simulink model "Controllo_assex_Rigido"  (R2020b)
settings: Solver=VariableStepAuto  StartTime=0.0  StopTime=5  RelTol=1e-3
values from neighbouring files (symbols this model uses):
  m = config_dc(parx)    [main.m]
  parx = parametri()    [main.m]
undefined symbols (not defined in the file or in its folder): Evaluate_Trajectory
libraries: cstblocks x2
settings Model: Creator=stefa  LastModifiedBy=user
settings DebuggingCC: AlgebraicLoopMsg=none  SFMachineParentedDataDiag=error

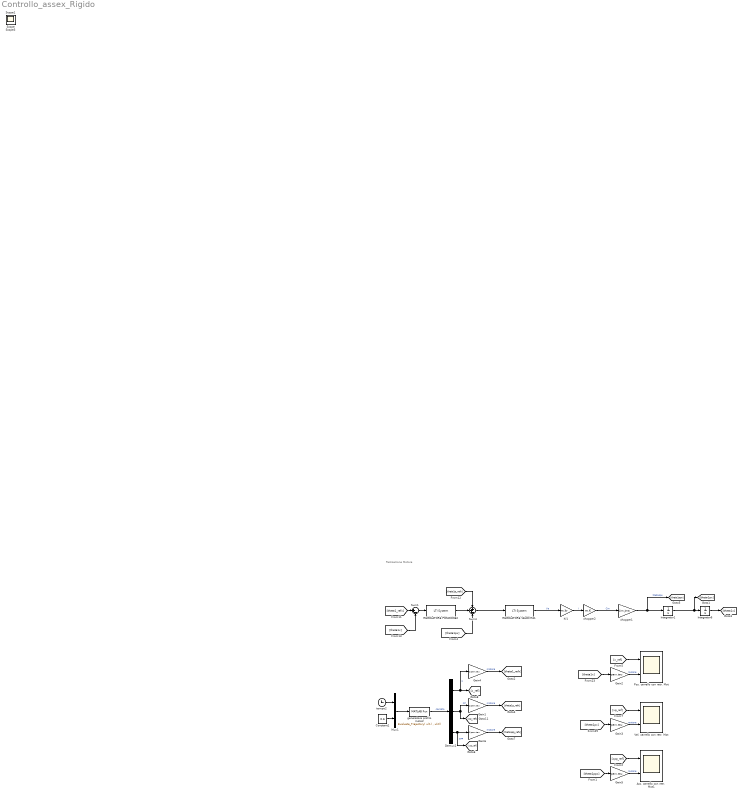
== system Controllo_assex_Rigido ==
  note: Retroazione Motore
  Acc. carrello con retr. Mot1 : Scope  NumInputPorts=2
  Constant1 : Constant  Value=0.6
  Demux2 : Demux  Outputs=3
  Gain1 : Gain  Gain=1/parx.tau
  Gain2 : Gain  Gain=parx.tau
  Gain3 : Gain  Gain=parx.tau
  Gain4 : Gain  Gain=1/parx.tau
  Gain5 : Gain  Gain=parx.tau
  Gain6 : Gain  Gain=1/parx.tau
  Integrator1 : Integrator
  Integrator6 : Integrator
  Kr1 : Gain  Gain=m.kr
  Mux1 : Mux  Inputs=2
  Pos. carrello con retr. Mot : Scope  NumInputPorts=2
  REGOLATORE POSIZIONE2 : cstblocks/LTI System  sys=ap.H_P  IC=[]
  REGOLATORE VELOCITA1 : cstblocks/LTI System  sys=av.PI_V  IC=[]
  Sum1 : Sum  Inputs=|+-
  Sum4 : Sum  Inputs=++-
  Vel. carrello con retr. Mot : Scope  NumInputPorts=2
  chopper1 : Gain  Gain=1/m.Jma
  chopper2 : Gain  Gain=m.K
  generatore profilo moto2 : MATLABFcn  MATLABFcn=Evaluate_Trajectory( u(1) , u(2))  OutputDimensions=3
  tempo2 : Clock
  Scope : Scope
  Scope1 : Scope
  Scope3 : Scope
  wires:
  Mux1/1 -> generatore profilo moto2/1
  generatore profilo moto2/1 -> Demux2/1  "carrello"
  Constant1/1 -> Mux1/2
  tempo2/1 -> Mux1/1
  Demux2/1 -> [x_ref], Gain4/1  "X"
  Demux2/2 -> Gain1/1, [xp_ref]  "XP"
  Kr1/1 -> chopper2/1  "I"
  Sum1/1 -> REGOLATORE POSIZIONE2/1
  REGOLATORE POSIZIONE2/1 -> Sum4/2
  REGOLATORE VELOCITA1/1 -> Kr1/1  "Va"
  [xp_ref] -> Vel. carrello con retr. Mot/1
  Sum4/1 -> REGOLATORE VELOCITA1/1
  [x_ref] -> Pos. carrello con retr. Mot/1
  [theta1p_refx] -> Sum4/1
  [theta1_refx] -> Sum1/1
  [theta1px] -> Sum4/3
  [theta1x] -> Sum1/2
  Gain1/1 -> [theta1p_refx]  "motore"
  Gain4/1 -> [theta1_refx]  "motore"
  chopper2/1 -> chopper1/1  "Cm"
  [theta1x] -> Gain2/1
  [theta1px] -> Gain3/1
  Gain3/1 -> Vel. carrello con retr. Mot/2  "motore"
  Gain2/1 -> Pos. carrello con retr. Mot/2  "motore"
  Integrator6/1 -> [theta1x]
  chopper1/1 -> [theta1ppx], Integrator1/1  "theta1px"
  Integrator1/1 -> [theta1px], Integrator6/1
  [theta1ppx] -> Gain5/1
  Gain5/1 -> Acc. carrello con retr. Mot1/2  "motore"
  [xpp_ref] -> Acc. carrello con retr. Mot1/1
  Demux2/3 -> Gain6/1, [xpp_ref]  "XPP"
  Gain6/1 -> [theta1pp_refx]  "motore"
